simulink model "GPS_test"  (Simulink 7.5)
settings: Solver=FixedStepDiscrete  SolverMode=SingleTasking  StartTime=0.0  StopTime=10.0  FixedStep=0.01  RelTol=1e-3
InitFcn:
  | boat_constants
undefined symbols (not defined in the file): cpInitCommunications, getGpsData, Init_onlyOnce, Init_Reset, initGps, processNewGpsData, T_step, u1, uart1EnqueueStateData, y1
libraries: dsPICdrivers x8, simulink x1
settings Model: Creator=Bryant Mairs  LastModifiedBy=Bryant
settings OptimizationCC: InlineParams=on  OptimizeModelRefInitCode=on  LifeSpan=1
settings HardwareCC: ProdBitPerInt=16  ProdEndianess=LittleEndian  ProdWordSize=16  ProdHWDeviceType=16-bit Generic
settings RTWCC: SystemTargetFile=dspic.tlc  MakeCommand=make_CreateMPLAB  TemplateMakefile=dspic_pic30_gcc.tmf  PostCodeGenCommand=dsPIC_Compile()  Description=Embedded Target for Microchip dsPIC (real-time)  ProcessScript=dspic_make_rtw_hook
settings RTWCC: CustomSource=|
  | circBuffer.c
  | ../../clib/conversions.c
  | ../../clib/gps.c
  | ../../clib/uart1.c
  | ../../clib/uart2.c
  | ../../clib/nmea0183.c
  | ../../clib/commProtocol.c
settings CodeAppCC: IgnoreCustomStorageClasses=off
settings STFCustomTargetCC: IncludeMdlTerminateFcn=off  CombineOutputUpdateFcns=on  SuppressErrorStatus=on  ERTCustomFileBanners=on  SupportContinuousTime=off  SupportNonInlinedSFcns=off  SystemTargetFile=dspic.tlc
settings ERTTargetCC: MultiwordLength=2048  ParMdlRefBuildCompliant=off  CompOptLevelCompliant=off  IncludeMdlTerminateFcn=off  SuppressErrorStatus=on  ERTFirstTimeCompliant=off  ModelStepFunctionPrototypeControlCompliant=off  CPPClassGenCompliant=off  ExtModeMexFile=ext_serial_win32_comm  InlinedParameterPlacement=NonHierarchical  ERTSrcFileBannerTemplate=dsPIC_code_template.cgt  ERTHdrFileBannerTemplate=dsPIC_code_template.cgt  ERTDataSrcFileTemplate=dsPIC_code_template.cgt  ERTDataHdrFileTemplate=dsPIC_code_template.cgt  ERTCustomFileTemplate=dsPIC_main.tlc  ConvertIfToSwitch=off
settings CustomProperty: DataType=string  Value=C:\PROGRA~1\MATLAB\R2010a\bin\win64\gmake

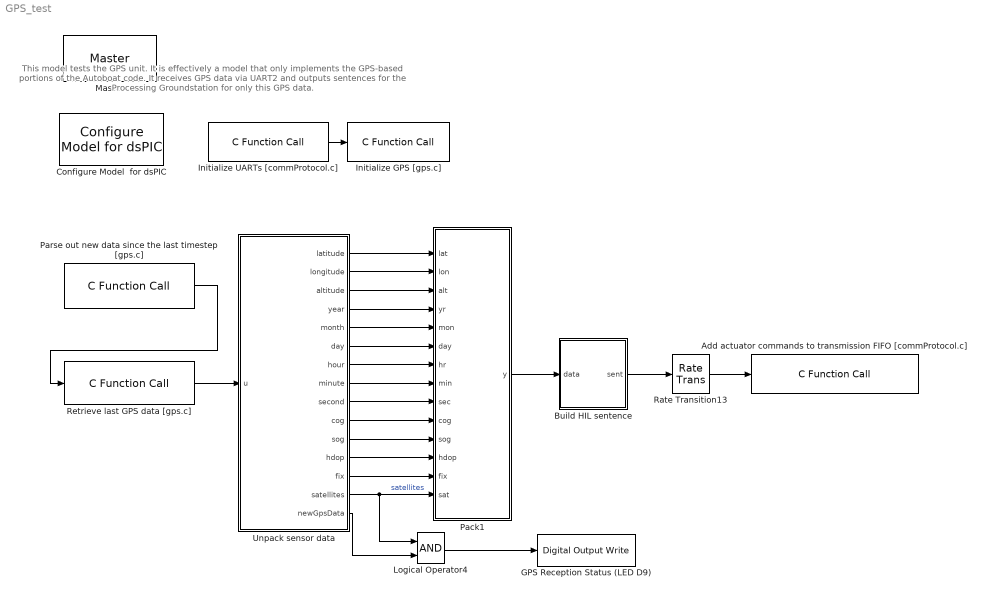
== system GPS_test ==
  note: This model tests the GPS unit. It is effectively
      | a model that only implements the GPS-based
      | portions of the Autoboat code. It receives GPS
      | data via UART2 and outputs sentences for the
      | Processing Groundstation for only this GPS data.
  Add actuator commands to transmission FIFO [commProtocol.c] : dsPICdrivers/OTHERS/C Function Call  Tag=dsPIC_dsPIC_CFunctionCall  FctUpdate=Output Function  fctName='uart1EnqueueStateData'  INPUT_SIZE=160  INPUT1=uint8  INPUT2=--  INPUT3=--  OUTPUT_SIZE=1  OUTPUT1=--  SampleTime=-1  InputType=[ 2 ]  OutputType=[ ]  FctDeclaration=extern void uart1EnqueueStateData(uint8_T* u1);  FctCall=uart1EnqueueStateData(*%u1);  OrderingInOutPopup=None  FctStart=None  FctStart_Name=Init_onlyOnce  FctStart_Declaration=inline extern void Init_onlyOnce();  FctStart_Call=Init_onlyOnce();  FctInit=None  FctInit_Name=Init_Reset  FctInit_Declaration=inline extern void Init_Reset();  FctInit_Call=Init_Reset();  PinDigitalInput=[]  PinDigitalOutput=[]  AnalogueInput=[]
  Build HIL sentence : Subsystem
  Configure Model  for dsPIC : dsPICdrivers/Simulink Configuration/Configure Model  for dsPIC
  GPS Reception Status (LED D9) : dsPICdrivers/Digital I//O/Digital Output Write  Tag=dsPIC_Digital_Output  Priority=5  PORT=A  Pin=[6]  Simultaneous=off  OrderingInOutPopup=None
  Initialize GPS [gps.c] : dsPICdrivers/OTHERS/C Function Call  Tag=dsPIC_dsPIC_CFunctionCall  FctUpdate=None  fctName='initGps'  INPUT_SIZE=1  INPUT1=--  INPUT2=--  INPUT3=--  OUTPUT_SIZE=1  OUTPUT1=--  SampleTime=Inf  InputType=[]  OutputType=[]  FctDeclaration=extern void initGps();  FctCall=initGps();  OrderingInOutPopup=Input  FctStart=Start Function (Call once and only once)  FctStart_Name=initGps  FctStart_Declaration=inline extern void initGps();  FctStart_Call=initGps();  FctInit=None  FctInit_Name=Init_Reset  FctInit_Declaration=inline extern void Init_Reset();  FctInit_Call=Init_Reset();  PinDigitalInput=[]  PinDigitalOutput=[]  AnalogueInput=[]
  Initialize UARTs [commProtocol.c] : dsPICdrivers/OTHERS/C Function Call  Tag=dsPIC_dsPIC_CFunctionCall  FctUpdate=None  fctName=cpInitCommunications  INPUT_SIZE=1  INPUT1=--  INPUT2=--  INPUT3=--  OUTPUT_SIZE=1  OUTPUT1=--  SampleTime=Inf  InputType=[]  OutputType=[]  FctDeclaration=extern void cpInitCommunications();  FctCall=cpInitCommunications();  OrderingInOutPopup=Output  FctStart=Start Function (Call once and only once)  FctStart_Name=cpInitCommunications  FctStart_Declaration=inline extern void cpInitCommunications();  FctStart_Call=cpInitCommunications();  FctInit=None  FctInit_Name=Init_Reset  FctInit_Declaration=inline extern void Init_Reset();  FctInit_Call=Init_Reset();  PinDigitalInput=[]  PinDigitalOutput=[]  AnalogueInput=[]
  Logical Operator4 : Logic  AllPortsSameDT=off  OutDataTypeMode=boolean  LogicDataType=fixdt(0, 8)  OutDataTypeStr=boolean
  Master : dsPICdrivers/Master  Tag=dsPIC_MASTER  Priority=1  TimeStepType=Timer1  picType=33fJ256GP710A  fcy=40000000  Quartz_33f=8e6  PLLActive_33f=on  fcyDesired_33f=40000000  tmr1="[8  49999  0]"  tmr1Info="Time Step : 0.01  ;   Error : 0%  PR1=49999"  tmr2345="[0  0  0  0  0  0  0  0]"  tmr2345cfg=[-1 -1 -1 -1 -1 -1 -1 -1]  IOautoConf=on  typePort="[ 0   0   0   0   0   0  10   0   0   0   0   0   0   0   0   0   0   0   0   0   0   0   0   0   0   0   0   0   0   0   0   0   0   0   0   0   0   0   0   0   0   0   0   0   0   0   0   0   0   0   0   0   0   0   0   0   0   0   0   0   0   0   0   0   0   0   0   0   0   0   0   0   0   0   0   0   0   0   0   0   0   0   0   0   0   0   0   0   0   0   0   0   0   0   0   0   0   0   0   0   0   0   0   0   0   0   0   0   0   0   0   0 ]"  TRIS="[ 65471  65535  65535  65535  65535  65535  65535 ]"  ADPCFG=4194304  MasterBusyPort=None  MasterOverloadPort=None  FOSC=Quartz (XT - HS)  ClockSwitchMonitor=Both disabled  TempProtection_33f=TEMP_ON  FPBOR=<empty>  PWRT=disable  MCLR=<empty>  ICD=ICS_PGD1  JTAGEN=JTAGEN_OFF  PowerSave=off  OverrideFcy=off  NewFcy=1e6  PR2345="[65535  65535  65535  65535  65535  65535  65535  65535]"
  Pack1 : Stateflow chart  TreatAsAtomicUnit=on
  Parse out new data since the last timestep [gps.c] : dsPICdrivers/OTHERS/C Function Call  Tag=dsPIC_dsPIC_CFunctionCall  FctUpdate=Output Function  fctName='processNewGpsData'  INPUT_SIZE=1  INPUT1=--  INPUT2=--  INPUT3=--  OUTPUT_SIZE=1  OUTPUT1=--  SampleTime=T_step  InputType=[ ]  OutputType=[ ]  FctDeclaration=extern void processNewGpsData();  FctCall=processNewGpsData();  OrderingInOutPopup=Output  FctStart=None  FctStart_Name=Init_onlyOnce  FctStart_Declaration=inline extern void Init_onlyOnce();  FctStart_Call=Init_onlyOnce();  FctInit=None  FctInit_Name=Init_Reset  FctInit_Declaration=inline extern void Init_Reset();  FctInit_Call=Init_Reset();  PinDigitalInput=[]  PinDigitalOutput=[]  AnalogueInput=[]
  Rate Transition13 : RateTransition  OutPortSampleTime=telemetryDataRate
  Retrieve last GPS data [gps.c] : dsPICdrivers/OTHERS/C Function Call  Tag=dsPIC_dsPIC_CFunctionCall  FctUpdate=Output Function  fctName='getGpsData'  INPUT_SIZE=1  INPUT1=--  INPUT2=--  INPUT3=--  OUTPUT_SIZE=33  OUTPUT1=uint8  SampleTime=T_step  InputType=[ ]  OutputType=[ 2 ]  FctDeclaration=extern void getGpsData(uint8_T* y1);  FctCall=getGpsData(*%y1);  OrderingInOutPopup=Input  FctStart=None  FctStart_Name=Init_onlyOnce  FctStart_Declaration=inline extern void Init_onlyOnce();  FctStart_Call=Init_onlyOnce();  FctInit=None  FctInit_Name=Init_Reset  FctInit_Declaration=inline extern void Init_Reset();  FctInit_Call=Init_Reset();  PinDigitalInput=[]  PinDigitalOutput=[]  AnalogueInput=[]
  Unpack sensor data : Stateflow chart  TreatAsAtomicUnit=on
  wires:
  Parse out new data since the last timestep [gps.c]/1 -> Retrieve last GPS data [gps.c]/1
  Retrieve last GPS data [gps.c]/1 -> Unpack sensor data/1(u)
  Initialize UARTs [commProtocol.c]/1 -> Initialize GPS [gps.c]/1
  Pack1/1(y) -> Build HIL sentence/1(data)
  Build HIL sentence/1(sent) -> Rate Transition13/1
  Unpack sensor data/1(latitude) -> Pack1/1(lat)
  Unpack sensor data/2(longitude) -> Pack1/2(lon)
  Unpack sensor data/3(altitude) -> Pack1/3(alt)
  Unpack sensor data/4(year) -> Pack1/4(yr)
  Unpack sensor data/5(month) -> Pack1/5(mon)
  Unpack sensor data/6(day) -> Pack1/6(day)
  Unpack sensor data/7(hour) -> Pack1/7(hr)
  Unpack sensor data/8(minute) -> Pack1/8(min)
  Unpack sensor data/9(second) -> Pack1/9(sec)
  Unpack sensor data/10(cog) -> Pack1/10(cog)
  Unpack sensor data/11(sog) -> Pack1/11(sog)
  Unpack sensor data/12(hdop) -> Pack1/12(hdop)
  Unpack sensor data/13(fix) -> Pack1/13(fix)
  Unpack sensor data/14(satellites) -> Pack1/14(sat), Logical Operator4/1  "satellites"
  Unpack sensor data/15(newGpsData) -> Logical Operator4/2
  Logical Operator4/1 -> GPS Reception Status (LED D9)/1
  Rate Transition13/1 -> Add actuator commands to transmission FIFO [commProtocol.c]/1

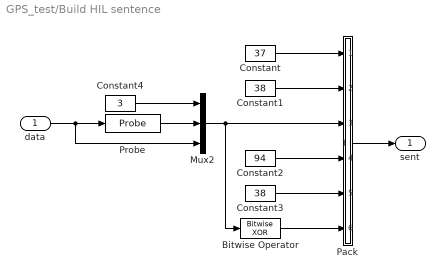
== system GPS_test/Build HIL sentence ==
  data : Inport
  Bitwise Operator : simulink/Logic and Bit Operations/Bitwise Operator  logicop=XOR  UseBitMask=off  BitMask=bin2dec('11011001')  BitMaskRealWorld=Stored Integer
  Constant : Constant  Value=37  OutDataTypeMode=uint8  OutDataType=fixdt(1, 16)  OutScaling=2^0  OutDataTypeStr=uint8
  Constant1 : Constant  Value=38  OutDataTypeMode=uint8  OutDataType=fixdt(1, 16)  OutScaling=2^0  OutDataTypeStr=uint8
  Constant2 : Constant  Value=94  OutDataTypeMode=uint8  OutDataType=fixdt(1, 16)  OutScaling=2^0  OutDataTypeStr=uint8
  Constant3 : Constant  Value=38  OutDataTypeMode=uint8  OutDataType=fixdt(1, 16)  OutScaling=2^0  OutDataTypeStr=uint8
  Constant4 : Constant  Value=3  OutDataTypeMode=uint8  OutDataType=fixdt(1, 16)  OutScaling=2^0  OutDataTypeStr=uint8
  Mux2 : Mux  Inputs=3
  Pack : Stateflow chart  TreatAsAtomicUnit=on
  Probe : Probe  ProbeSampleTime=off  ProbeComplexSignal=off  ProbeWidthDataType=uint8
  sent : Outport
  wires:
  data/1 -> Probe/1, Mux2/3
  Constant/1 -> Pack/1(a)
  Constant1/1 -> Pack/2(b)
  Pack/1(y) -> sent/1
  Mux2/1 -> Bitwise Operator/1, Pack/3(c)
  Probe/1 -> Mux2/2
  Constant2/1 -> Pack/4(d)
  Constant3/1 -> Pack/5(e)
  Bitwise Operator/1 -> Pack/6(f)
  Constant4/1 -> Mux2/1

== matlab function Unpack sensor data ==
  data: latitude output double; longitude output double; altitude output double; year output double; month output double; day output double; hour output double; minute output double; second output double; cog output double; sog output double; u input uint8; hdop output double; fix output double; satellites output double; newGpsData output double
function [latitude, longitude, altitude, year, month, day, hour, minute, second, cog, sog, hdop, fix, satellites, newGpsData] = unpack(u)
%#eml

latitude = typecast(u(1:4), 'single');
longitude = typecast(u(5:8), 'single');
altitude = typecast(u(9:12), 'single');
year = u(13);
month = u(14);
day = u(15);
hour = u(16);
minute = u(17);
second = u(18);
cog = typecast(u(19:22), 'single');
sog = typecast(u(23:26), 'single');
hdop = typecast(u(27:30), 'single');
fix = u(31);
satellites = u(32);
newGpsData = u(33);

== matlab function Pack1 ==
  data: y output double; lat input double; lon input double; alt input double; yr input double; mon input double; day input double; hr input double; min input double; sec input double; cog input double; sog input double; hdop input double; fix input double; sat input double
function y = fcn(lat, lon, alt, yr, mon, day, hr, min, sec, cog, sog, hdop, fix, sat)
%#eml

y = zeros(153, 1, 'uint8');
y(57:60) = packUint32BE(typecast(lat,'uint32'));
y(61:64) = packUint32BE(typecast(lon,'uint32'));
y(65:68) = packUint32BE(typecast(alt,'uint32'));
y(69) = yr;
y(70) = mon;
y(71) = day;
y(72) = hr;
y(73) = min;
y(74) = sec;
y(75:78) = packUint32BE(typecast(cog,'uint32'));
y(79:82) = packUint32BE(typecast(sog,'uint32'));
y(83:86) = packUint32BE(typecast(hdop,'uint32'));
y(87) = fix;
y(88) = sat;

function out = packUint32BE(in)
out = zeros(4, 1, 'uint8');
out(1) = uint8(bitand(bitshift(in,-24),hex2dec('FF')));
out(2) = uint8(bitand(bitshift(in,-16),hex2dec('FF')));
out(3) = uint8(bitand(bitshift(in,-8),hex2dec('FF')));
out(4) = uint8(bitand(in,hex2dec('FF')));

== matlab function Build HIL sentence/Pack ==
  data: a input double; y output double; b input double; c input double; d input double; e input double; f input double
function y = fcn(a, b, c, d, e, f)
%#eml

y = zeros(length(a)+length(b)+length(c)+length(d)+length(e)+length(f), 1, 'uint8');
y(1) = a;
y(2) = b;
y(3:157) = c;
y(158) = d;
y(159) = e;
y(160) = f;
